simulink model "Lab7__SinglePhaseInvertorQuasiSquareWave"  (R2021a)
settings: Solver=VariableStepAuto  StartTime=0.0  StopTime=0.1  RelTol=1e-3
libraries: spsIGBTDiodeLib x4, spsCurrentMeasurementLib x1, spsDCVoltageSourceLib x1, spsRMSLib x1, spsSeriesRLCBranchLib x1, spsVoltageMeasurementLib x1, spspowerguiLib x1
settings Model: Creator=Prabhav Shah  LastModifiedBy=hp

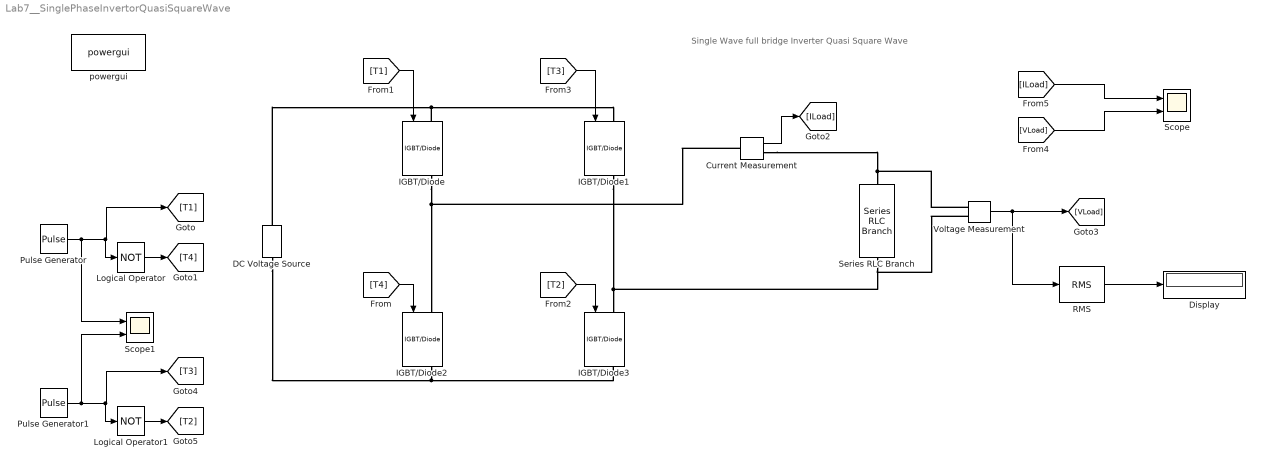
== system Lab7__SinglePhaseInvertorQuasiSquareWave ==
  note: Single Wave full bridge Inverter Quasi Square Wave
  Current Measurement : spsCurrentMeasurementLib/Current Measurement  PhasorSimulation=off  OutputType=Complex  PSBequivalent=0
  DC Voltage Source : spsDCVoltageSourceLib/DC Voltage Source  Amplitude=100  Measurements=None
  Display : Display
  IGBT/Diode{,1..3} (4 alike) : spsIGBTDiodeLib/IGBT//Diode  Ron=1e-3  Rs=1e5  Cs=inf  Measurements=on
  Logical Operator : Logic  Operator=NOT  AllPortsSameDT=off  OutDataTypeStr=boolean
  Logical Operator1 : Logic  Operator=NOT  AllPortsSameDT=off  OutDataTypeStr=boolean
  Pulse Generator : DiscretePulseGenerator  PulseType=Time based  Period=0.02  PulseWidth=50  PhaseDelay=(0.02/360)*45
  Pulse Generator1 : DiscretePulseGenerator  PulseType=Time based  Period=0.02  PulseWidth=25  PhaseDelay=225/360*0.02
  RMS : spsRMSLib/RMS  TrueRMS=on  Freq=60  RMSInit=120  Ts=0
  Scope : Scope  NumInputPorts=2
  Scope1 : Scope  NumInputPorts=2
  Series RLC Branch : spsSeriesRLCBranchLib/Series RLC Branch  LConnTagsString=__new0  RConnTagsString=__new0  BranchType=R  Resistance=10  Inductance=1e-3  SetiL0=off  InitialCurrent=0  Capacitance=1e-6  Setx0=off  InitialVoltage=0  Measurements=None
  Voltage Measurement : spsVoltageMeasurementLib/Voltage Measurement  PhasorSimulation=off  OutputType=Complex  PSBequivalent=0
  powergui : spspowerguiLib/powergui  Priority=1  SimulationMode=Discrete  SampleTime=50e-6  frequency=60  Iterations=50  frequencyindice=0  Pbase=100e6  ErrMax=1e-4  UnitsV=kV  UnitsW=MW  buscounter=0  FunctionMessages=off  echomessages=off  EnableUseOfTLC=off  CurrentSourceSwitches=off  DisableSnubberDevices=off  DisableRonSwitches=off  DisableVfSwitches=off  DisplayEquations=off  AutomaticDiscreteSolvers=off  SolverType=Tustin/Backward Euler (TBE)  Interpol=off  ExternalGateDelay=off  methode=off  Ts=100  x0status=blocks  SPID=on  SwTol=0  HookPort=off  NonlinearTolerance=1e-4  nMaxIteration=100  ContinueOnMaxIteration=off  RestoreLinks=warning  ResistiveCurrentMeasurement=off  Frange=[0:2:500]  Ylog=off  Xlog=on  ShowGrid=off  save=off  variable=ZData  structure=0  ZoomFFT=off  StartTime=0.0  cycles=1  DisplayStyle=1  fundamental=60  FreqAxis=off  MaxFrequency=1000  frequencyindicesteady=1  RmsSteady=1  display=off
  wires:
  Pulse Generator/1 -> Scope1/1, Logical Operator/1, [T1]
  Logical Operator/1 -> [T4]
  [T1] -> IGBT/Diode/1
  [T3] -> IGBT/Diode1/1
  [T4] -> IGBT/Diode2/1
  [T2] -> IGBT/Diode3/1
  Current Measurement/1 -> [ILoad]
  Voltage Measurement/1 -> RMS/1, [VLoad]
  RMS/1 -> Display/1
  [ILoad] -> Scope/1
  [VLoad] -> Scope/2
  Logical Operator1/1 -> [T2]
  Pulse Generator1/1 -> Scope1/2, Logical Operator1/1, [T3]
  connections:
  DC Voltage Source/RConn1 -- IGBT/Diode/LConn1 -- IGBT/Diode1/LConn1
  DC Voltage Source/LConn1 -- IGBT/Diode2/RConn1 -- IGBT/Diode3/RConn1
  IGBT/Diode/RConn1 -- Current Measurement/LConn1 -- IGBT/Diode2/LConn1
  IGBT/Diode1/RConn1 -- Voltage Measurement/LConn2 -- Series RLC Branch/RConn1 -- IGBT/Diode3/LConn1
  Current Measurement/RConn1 -- Voltage Measurement/LConn1 -- Series RLC Branch/LConn1
